simulink model "sampleModel1611"  (R2023a)
settings: Solver=VariableStepAuto  StartTime=0.0  StopTime=10.0  RelTol=1e-3
libraries: simulink x4
settings Model: Creator=user1  LastModifiedBy=user1

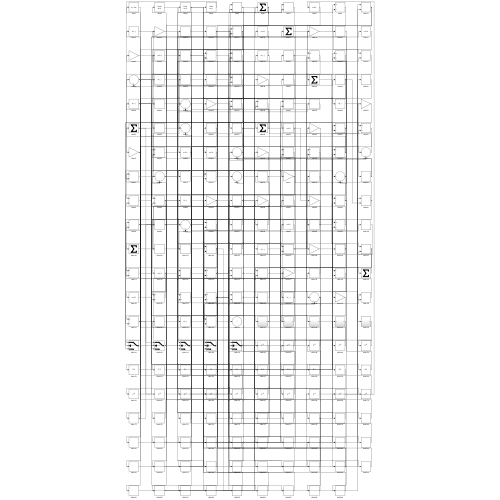
[thumbnail: Simulink's stored preview of the top-level diagram]
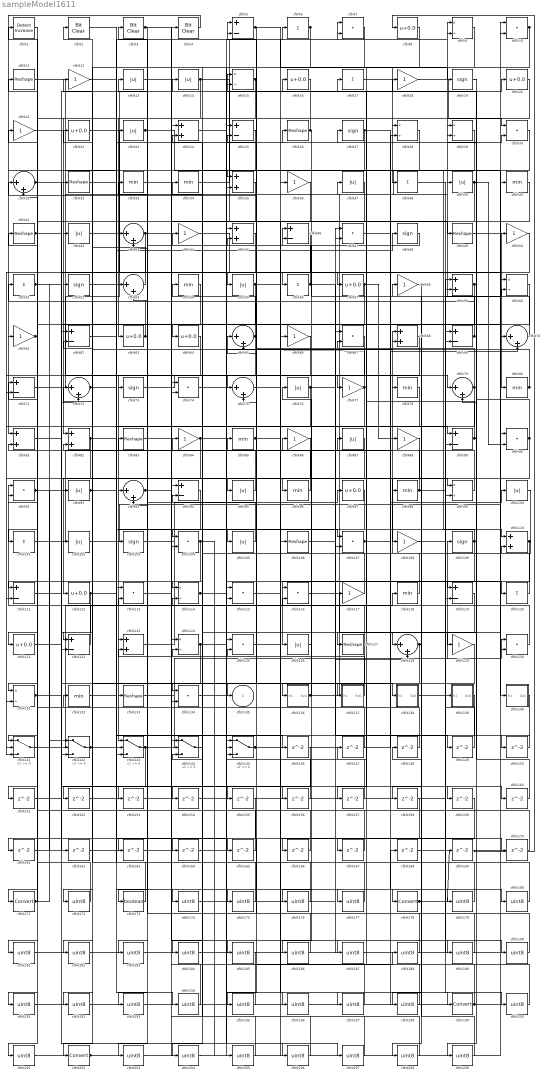
== system sampleModel1611 ==
  cfblk1 : simulink/Logic and Bit Operations/Detect Increase  vinit=0.0  OutDataTypeStr=boolean
      settings: LibrarySourceBlock=|
      | hdlsllib/Logic and Bit
      | Operations/Detect
      | Increase
  cfblk{7,10,30,47,67,74,90..91,104,107,113,115..116,125,130,134} (16 alike) : DotProduct  OutDataTypeStr=Inherit: Inherit via internal rule
  cfblk{13..14,23,37,39,42,55,76,87,92,95,100,102,105,126} (15 alike) : Abs  SaturateOnIntegerOverflow=off
  cfblk{6,17,38,51,56,101,120} (7 alike) : Sum  Inputs=+
  cfblk{19,27,48,52,73,103,109} (7 alike) : Signum
  cfblk{11,26,32,41,49,83,106,127,133} (9 alike) : Reshape
  cfblk{12,18,21,36,44,50,58,61,66,77,84,86,88,108,117,129} (16 alike) : Gain
  cfblk{24,35,45,59,68,81..82,110,123} (9 alike) : Sum
  cfblk{5,25,46,62,69,71,89,94,111,119,122} (11 alike) : Sum  Inputs=+-
  cfblk{8,16,20,22,57,63..64,97,112,121} (10 alike) : Bias  Bias=0.0  SaturateOnIntegerOverflow=off
  cfblk{9,15,28..29,60,99,114,124,131} (9 alike) : Product  Inputs=*/  RndMeth=Zero  SaturateOnIntegerOverflow=on
  cfblk{33..34,40,54,78,80,85,96,98,118,132} (11 alike) : MinMax
  cfblk{31,43,53,65,70,72,75,79,93,128} (10 alike) : Sum  Inputs=|++
  cfblk136 : Subsystem
      settings: LibrarySourceBlock=|
      | hdlsllib/Ports &
      | Subsystems/Subsystem
  cfblk137 : Subsystem
      settings: LibrarySourceBlock=|
      | hdlsllib/Ports &
      | Subsystems/Subsystem
  cfblk138 : Subsystem
      settings: LibrarySourceBlock=|
      | hdlsllib/Ports &
      | Subsystems/Subsystem
  cfblk139 : Subsystem
      settings: LibrarySourceBlock=|
      | hdlsllib/Ports &
      | Subsystems/Subsystem
  cfblk140 : Subsystem
      settings: LibrarySourceBlock=|
      | hdlsllib/Ports &
      | Subsystems/Subsystem
  cfblk{141..145} (5 alike) : Switch  SaturateOnIntegerOverflow=off  InputSameDT=off
  cfblk{146..170} (25 alike) : Delay  SampleTime=1
  cfblk{171,178,199,202} (4 alike) : DataTypeConversion  SaturateOnIntegerOverflow=off  RndMeth=Floor
  cfblk{172,174..177,179..198,200..201,203..209} (34 alike) : DataTypeConversion  OutDataTypeStr=uint8  SaturateOnIntegerOverflow=off  RndMeth=Floor
  cfblk173 : DataTypeConversion  OutDataTypeStr=boolean  SaturateOnIntegerOverflow=off  RndMeth=Floor
  cfblk2 : simulink/Logic and Bit Operations/Bit Clear  iBit=0
      settings: LibrarySourceBlock=|
      | hdlsllib/Logic and Bit
      | Operations/Bit Clear
  cfblk3 : simulink/Logic and Bit Operations/Bit Clear  iBit=0
      settings: LibrarySourceBlock=|
      | hdlsllib/Logic and Bit
      | Operations/Bit Clear
  cfblk4 : simulink/Logic and Bit Operations/Bit Clear  iBit=0
      settings: LibrarySourceBlock=|
      | hdlsllib/Logic and Bit
      | Operations/Bit Clear
  cfblk135 : Outport  VectorParamsAs1DForOutWhenUnconnected=off
  wires:
  cfblk141/1 -> cfblk118/1
  cfblk70/1 -> cfblk9/1
  cfblk66/1 -> cfblk75/1
  cfblk116/1 -> cfblk128/1
  cfblk65/1 -> cfblk54/1, cfblk142/2
  cfblk133/1 -> cfblk109/1
  cfblk34/1 -> cfblk6/1
  cfblk64/1 -> cfblk143/1
  cfblk31/1 -> cfblk110/1, cfblk138/1(In1), cfblk159/1
  cfblk136/1(Out1) -> cfblk39/1, cfblk116/2
  cfblk118/1 -> cfblk68/1
  cfblk11/1 -> cfblk77/1
  cfblk84/1 -> cfblk123/1, cfblk189/1
  cfblk92/1 -> cfblk9/2, cfblk194/1
  cfblk19/1 -> cfblk129/1
  cfblk127/1 -> cfblk43/2, cfblk62/2, cfblk173/1
  cfblk108/1 -> cfblk69/1
  cfblk63/1 -> cfblk133/1, cfblk31/2, cfblk203/1
  cfblk123/1 -> cfblk97/1
  cfblk27/1 -> cfblk82/1, cfblk130/2
  cfblk95/1 -> cfblk34/1
  cfblk81/1 -> cfblk16/1
  cfblk56/1 -> cfblk3/1, cfblk120/1
  cfblk143/1 -> cfblk130/1, cfblk152/1
  cfblk6/1 -> cfblk75/2, cfblk145/3
  cfblk89/1 -> cfblk17/1, cfblk209/1
  cfblk20/1 -> cfblk63/1
  cfblk16/1 -> cfblk32/1
  cfblk17/1 -> cfblk38/1
  cfblk90/1 -> cfblk108/1, cfblk15/1
  cfblk91/1 -> cfblk86/1, cfblk206/1
  cfblk101/1 -> cfblk78/1
  cfblk128/1 -> cfblk157/1, cfblk158/1
  cfblk22/1 -> cfblk56/1
  cfblk100/1 -> cfblk110/2
  cfblk10/1 -> cfblk42/1, cfblk127/1
  cfblk120/1 -> cfblk44/1
  cfblk78/1 -> cfblk96/1
  cfblk52/1 -> cfblk37/1
  cfblk15/1 -> cfblk52/1, cfblk104/2
  cfblk126/1 -> cfblk76/1
  cfblk88/1 -> cfblk93/1
  cfblk18/1 -> cfblk30/1
  cfblk14/1 -> cfblk106/1, cfblk140/1(In1), cfblk151/1
  cfblk129/1 -> cfblk137/1(In1)
  cfblk75/1 -> cfblk30/2
  cfblk9/1 -> cfblk28/1
  cfblk80/1 -> cfblk12/1, cfblk25/2
  cfblk29/1 -> cfblk105/1
  cfblk71/1 -> cfblk14/1
  cfblk4/1 -> cfblk81/1
  cfblk54/1 -> cfblk121/1
  cfblk122/1 -> cfblk91/1
  cfblk105/1 -> cfblk33/1
  cfblk8/1 -> cfblk134/1
  cfblk5/1 -> cfblk135/1, cfblk19/1
  cfblk117/1 -> cfblk85/1
  cfblk131/1 -> cfblk18/1, cfblk162/1
  cfblk73/1 -> cfblk79/1
  cfblk55/1 -> cfblk7/2, cfblk170/1, cfblk191/1
  cfblk21/1 -> cfblk53/1
  cfblk7/1 -> cfblk95/1
  cfblk46/1 -> cfblk64/1
  cfblk124/1 -> cfblk87/1, cfblk7/1, cfblk192/1, cfblk207/1
  cfblk36/1 -> cfblk202/1
  cfblk86/1 -> cfblk112/1
  cfblk51/1 -> cfblk99/1, cfblk142/1
  cfblk87/1 -> cfblk102/1
  cfblk13/1 -> cfblk4/1
  cfblk82/1 -> cfblk89/1, cfblk20/1, cfblk131/2
  cfblk104/1 -> cfblk111/1, cfblk205/1
  cfblk107/1 -> cfblk100/1, cfblk70/2
  cfblk3/1 -> cfblk98/1, cfblk156/1, cfblk163/1
  cfblk110/1 -> cfblk126/1, cfblk116/1
  cfblk109/1 -> cfblk104/1, cfblk176/1
  cfblk30/1 -> cfblk79/2
  cfblk96/1 -> cfblk53/2
  cfblk69/1 -> cfblk46/1, cfblk51/1
  cfblk103/1 -> cfblk107/1
  cfblk50/1 -> cfblk111/2
  cfblk72/1 -> cfblk43/1, cfblk107/2
  cfblk61/1 -> cfblk141/1, cfblk21/1
  cfblk111/1 -> cfblk62/1
  cfblk53/1 -> cfblk22/1
  cfblk33/1 -> cfblk49/1
  cfblk32/1 -> cfblk26/1
  cfblk76/1 -> cfblk128/2, cfblk141/3
  cfblk49/1 -> cfblk80/1
  cfblk112/1 -> cfblk27/1, cfblk142/3
  cfblk60/1 -> cfblk73/1
  cfblk145/1 -> cfblk28/2, cfblk167/1
  cfblk93/1 -> cfblk5/1, cfblk155/1
  cfblk142/1 -> cfblk72/1, cfblk48/1
  cfblk1/1 -> cfblk171/1
  cfblk132/1 -> cfblk178/1
  cfblk102/1 -> cfblk90/1
  cfblk41/1 -> cfblk55/1, cfblk136/1(In1), cfblk70/1
  cfblk137/1(Out1) -> cfblk13/1
  cfblk130/1 -> cfblk71/1
  cfblk43/1 -> cfblk57/1, cfblk141/2
  cfblk59/1 -> cfblk29/1, cfblk119/2
  cfblk23/1 -> cfblk35/1, cfblk15/2
  cfblk37/1 -> cfblk114/1
  cfblk39/1 -> cfblk103/1, cfblk90/2, cfblk134/2
  cfblk35/1 -> cfblk101/1
  cfblk77/1 -> cfblk143/3, cfblk65/2, cfblk153/1
  cfblk44/1 -> cfblk60/1
  cfblk48/1 -> cfblk46/2
  cfblk68/1 -> cfblk71/2
  cfblk99/1 -> cfblk11/1
  cfblk114/1 -> cfblk68/2, cfblk119/1
  cfblk98/1 -> cfblk45/2, cfblk60/2
  cfblk115/1 -> cfblk199/1
  cfblk67/1 -> cfblk122/1
  cfblk57/1 -> cfblk93/2, cfblk88/1
  cfblk85/1 -> cfblk177/1, cfblk197/1
  cfblk42/1 -> cfblk59/2
  cfblk28/1 -> cfblk61/1
  cfblk26/1 -> cfblk23/1, cfblk166/1
  cfblk45/1 -> cfblk131/1
  cfblk79/1 -> cfblk31/1, cfblk161/1
  cfblk12/1 -> cfblk146/1
  cfblk147/1 -> cfblk91/2
  cfblk148/1 -> cfblk67/1
  cfblk106/1 -> cfblk149/1
  cfblk149/1 -> cfblk59/1
  cfblk140/1(Out1) -> cfblk150/1
  cfblk150/1 -> cfblk143/2
  cfblk151/1 -> cfblk122/2
  cfblk152/1 -> cfblk89/2
  cfblk153/1 -> cfblk69/2
  cfblk121/1 -> cfblk154/1
  cfblk154/1 -> cfblk99/2
  cfblk156/1 -> cfblk65/1
  cfblk157/1 -> cfblk45/1
  cfblk138/1(Out1) -> cfblk160/1
  cfblk160/1 -> cfblk29/2
  cfblk161/1 -> cfblk72/2
  cfblk162/1 -> cfblk25/1
  cfblk163/1 -> cfblk35/2
  cfblk119/1 -> cfblk164/1
  cfblk164/1 -> cfblk114/2
  cfblk62/1 -> cfblk165/1
  cfblk165/1 -> cfblk123/2
  cfblk166/1 -> cfblk5/2
  cfblk167/1 -> cfblk82/2
  cfblk168/1 -> cfblk10/2
  cfblk169/1 -> cfblk8/1
  cfblk170/1 -> cfblk41/1
  cfblk171/1 -> cfblk81/2, cfblk92/1
  cfblk146/1 -> cfblk172/1
  cfblk172/1 -> cfblk1/1
  cfblk173/1 -> cfblk2/1
  cfblk2/1 -> cfblk174/1
  cfblk174/1 -> cfblk117/1
  cfblk113/1 -> cfblk175/1
  cfblk175/1 -> cfblk145/2
  cfblk176/1 -> cfblk113/1
  cfblk177/1 -> cfblk113/2
  cfblk178/1 -> cfblk169/1, cfblk198/1
  cfblk134/1 -> cfblk179/1
  cfblk179/1 -> cfblk132/1
  cfblk47/1 -> cfblk180/1
  cfblk180/1 -> cfblk84/1
  cfblk25/1 -> cfblk181/1
  cfblk181/1 -> cfblk47/1
  cfblk155/1 -> cfblk182/1
  cfblk182/1 -> cfblk47/2
  cfblk40/1 -> cfblk183/1
  cfblk183/1 -> cfblk139/1(In1)
  cfblk97/1 -> cfblk184/1
  cfblk184/1 -> cfblk40/1
  cfblk83/1 -> cfblk185/1
  cfblk139/1(Out1) -> cfblk186/1
  cfblk186/1 -> cfblk83/1
  cfblk125/1 -> cfblk187/1
  cfblk187/1 -> cfblk67/2
  cfblk185/1 -> cfblk188/1
  cfblk188/1 -> cfblk125/1
  cfblk189/1 -> cfblk125/2
  cfblk74/1 -> cfblk190/1
  cfblk190/1 -> cfblk148/1
  cfblk191/1 -> cfblk74/1
  cfblk192/1 -> cfblk74/2
  cfblk94/1 -> cfblk193/1
  cfblk193/1 -> cfblk10/1
  cfblk194/1 -> cfblk94/1
  cfblk158/1 -> cfblk195/1
  cfblk195/1 -> cfblk94/2
  cfblk24/1 -> cfblk196/1
  cfblk196/1 -> cfblk168/1
  cfblk197/1 -> cfblk24/1
  cfblk198/1 -> cfblk24/2
  cfblk199/1 -> cfblk147/1, cfblk124/2
  cfblk38/1 -> cfblk200/1
  cfblk200/1 -> cfblk115/1
  cfblk159/1 -> cfblk201/1
  cfblk201/1 -> cfblk115/2
  cfblk202/1 -> cfblk50/1, cfblk124/1
  cfblk203/1 -> cfblk36/1
  cfblk144/1 -> cfblk204/1
  cfblk204/1 -> cfblk66/1
  cfblk205/1 -> cfblk144/1
  cfblk206/1 -> cfblk144/2
  cfblk207/1 -> cfblk144/3
  cfblk58/1 -> cfblk208/1
  cfblk208/1 -> cfblk145/1
  cfblk209/1 -> cfblk58/1

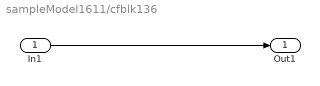
== system sampleModel1611/cfblk136 ==
  In1 : Inport
  Out1 : Outport
  wires:
  In1/1 -> Out1/1

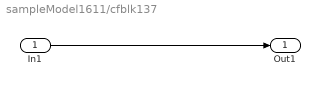
== system sampleModel1611/cfblk137 ==
  In1 : Inport
  Out1 : Outport
  wires:
  In1/1 -> Out1/1

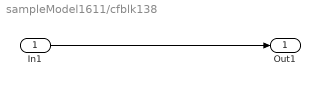
== system sampleModel1611/cfblk138 ==
  In1 : Inport
  Out1 : Outport
  wires:
  In1/1 -> Out1/1

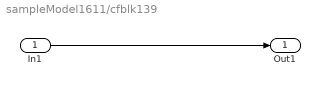
== system sampleModel1611/cfblk139 ==
  In1 : Inport
  Out1 : Outport
  wires:
  In1/1 -> Out1/1

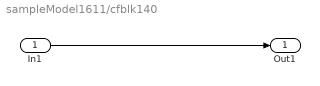
== system sampleModel1611/cfblk140 ==
  In1 : Inport
  Out1 : Outport
  wires:
  In1/1 -> Out1/1
